simulink model "Systemidentifikation"  (R2023b)
settings: Solver=ode5  StartTime=0.0  StopTime=10  MaxStep=1  RelTol=1e-3  AbsTol=1e-3
undefined symbols (not defined in the file or in its folder): stepFinalValue
libraries: Plants x1, softHIL x1
settings Model: Creator=mkottman  LastModifiedBy=Alex
settings SolverCC: AutoScaleAbsTol=off  AlgebraicLoopSolver=TrustRegion
settings DataIOCC: SaveFormat=Array  SignalLoggingSaveFormat=ModelDataLogs  SaveOutput=off  SaveTime=off  ReturnWorkspaceOutputs=off
settings OptimizationCC: BooleanDataType=off  ExpressionDepthLimit=2147483647  InitFltsAndDblsToZero=on  LifeSpan=inf
settings DebuggingCC: SaveWithParameterizedLinksMsg=none  UnderspecifiedInitializationDetection=Classic  MergeDetectMultiDrivingBlocksExec=none  SignalResolutionControl=TryResolveAllWithWarning  MultiTaskDSMMsg=warning  MultiTaskCondExecSysMsg=none  FcnCallInpInsideContextMsg=warning  UnconnectedInputMsg=warning  UnconnectedOutputMsg=warning  UnconnectedLineMsg=warning  StateNameClashWarn=warning  SFUnexpectedBacktrackingDiag=warning  SFNoUnconditionalDefaultTransitionDiag=warning  SFExecutionAtInitializationDiag=none  ArithmeticOperatorsInVariantConditions=warning
settings HardwareCC: ProdBitPerPointer=32  ProdBitPerSizeT=32  ProdBitPerPtrDiffT=32  ProdLargestAtomicFloat=None  ProdIntDivRoundTo=Undefined  ProdEndianess=Unspecified  ProdWordSize=32  ProdHWDeviceType=32-bit Generic  TargetUnknown=on
settings ModelReferenceCC: EnableRefExpFcnMdlSchedulingChecks=on  PropagateSignalLabelsOutOfModel=off
settings SFSimCC: SimUseLocalCustomCode=off  CustomCodeUndefinedFunction=UseInterfaceOnly
settings RTWCC: TemplateMakefile=grt_vc.tmf  RTWUseLocalCustomCode=off
settings CodeAppCC: StateflowObjectComments=on
settings GRTTargetCC: TargetFcnLib=ansi_tfl_tmw.mat  TargetLangStandard=C89/C90 (ANSI)  CombineOutputUpdateFcns=off  GRTInterface=on
settings ConfigComp: CovMetricSettings=dw  CovSaveCumulativeToWorkspaceVar=on  CovSaveSingleToWorkspaceVar=on  CovExternalEMLEnable=off

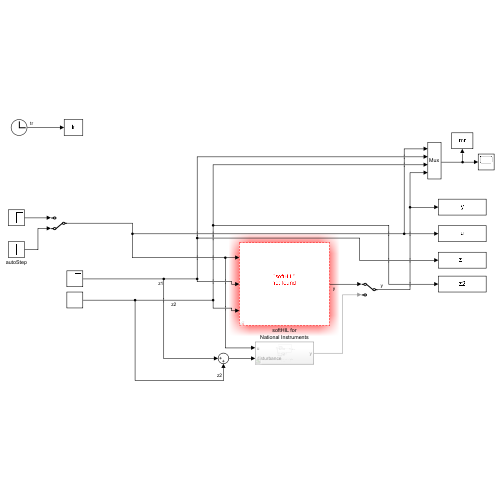
[thumbnail: Simulink's stored preview of the top-level diagram]
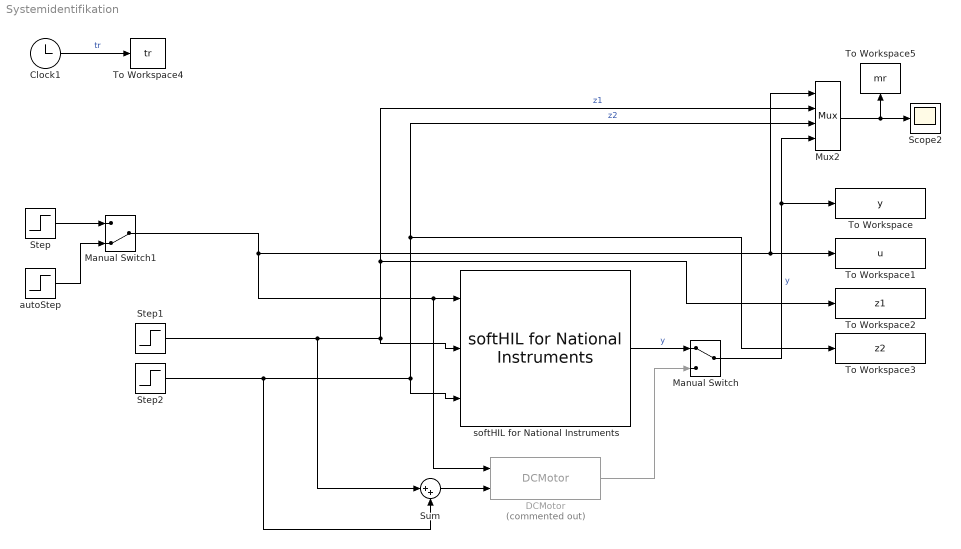
== system Systemidentifikation ==
  Clock1 : Clock
  DCMotor : Plants/DCMotor  Commented=on  SystemSampleTime=-1  VariantActivationTime=update diagram  AllowFlexibleInterface=on  Latency=0  AutoFrameSizeCalculation=off
  Manual Switch : ManualSwitch
  Manual Switch1 : ManualSwitch  CurrentSetting=0
  Mux2 : Mux
  Scope2 : Scope
  Step : Step  After=10  SampleTime=0.01
  Step1 : Step  Time=4  SampleTime=0.01
  Step2 : Step  Time=7  SampleTime=0.01
  Sum : Sum  Inputs=|++
  To Workspace : ToWorkspace  VariableName=y  SaveFormat=Timeseries  SampleTime=0.01
  To Workspace1 : ToWorkspace  VariableName=u  SaveFormat=Timeseries  SampleTime=0.01
  To Workspace2 : ToWorkspace  VariableName=z1  SaveFormat=Timeseries  SampleTime=0.01
  To Workspace3 : ToWorkspace  VariableName=z2  SaveFormat=Timeseries  SampleTime=0.01
  To Workspace4 : ToWorkspace  VariableName=tr  SampleTime=5/1000
  To Workspace5 : ToWorkspace  VariableName=mr  SampleTime=5/1000
  autoStep : Step  After=stepFinalValue  SampleTime=0.01
  softHIL for National Instruments : softHIL/softHIL for National Instruments  nAIn=1  nAOut=1  nDIn=0  nDOut=2  Sampletime=0.01  Servername=getservername  ServerOL=off  ClientOL=off  Delay=off
  wires:
  Clock1/1 -> To Workspace4/1  "tr"
  Mux2/1 -> Scope2/1, To Workspace5/1
  Manual Switch/1 -> To Workspace/1, Mux2/4  "y"
  Step1/1 -> Sum/1, softHIL for National Instruments/2, To Workspace2/1, Mux2/2  "z1"
  Step2/1 -> Sum/2, softHIL for National Instruments/3, To Workspace3/1, Mux2/3  "z2"
  Manual Switch1/1 -> Mux2/1, To Workspace1/1, DCMotor/1, softHIL for National Instruments/1
  softHIL for National Instruments/1 -> Manual Switch/1  "y"
  DCMotor/1 -> Manual Switch/2
  Step/1 -> Manual Switch1/1
  autoStep/1 -> Manual Switch1/2
  Sum/1 -> DCMotor/2
